simulink model "shaper_wok"  (R2020a)
settings: Solver=VariableStepAuto  StartTime=0.0  StopTime=100  RelTol=1e-3
settings Model: Creator=joshi  LastModifiedBy=joshi

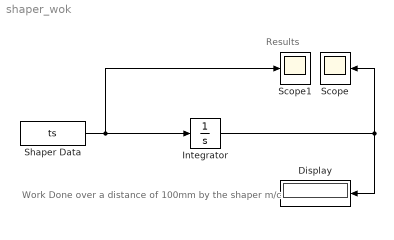
== system shaper_wok ==
  note: Work Done over a distance of 100mm by the shaper m/c
  note: Results
  Display : Display
  Integrator : Integrator
  Scope : Scope
  Scope1 : Scope
  Shaper Data : FromWorkspace  VariableName=ts
  wires:
  Shaper Data/1 -> Integrator/1, Scope1/1
  Integrator/1 -> Scope/1, Display/1
